simulink library "HWController_NGCHP_Genset_3p5MVA_lib"  (Simulink 8.1)
settings: Solver=ode45  StartTime=0.0  StopTime=10.0  RelTol=1e-3
undefined symbols (not defined in the file): Ts
libraries: HWController_NGCHP_Genset_3p5MVA_lib x2, powerlib x2, CHP_Model_lib x1, rtio_generic_modbus x1, simulink x1, GEJenbacherJ620_lib x1
settings Model: Creator=RE25624  LastModifiedBy=RE25624

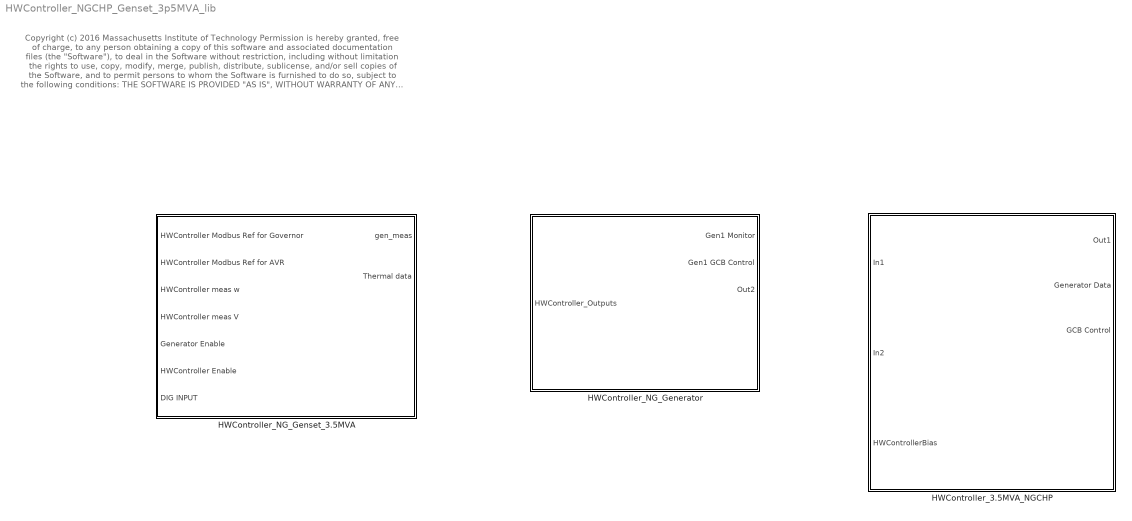
== system HWController_NGCHP_Genset_3p5MVA_lib ==
  note: Copyright (c) 2016 Massachusetts Institute of Technology
      | Permission is hereby granted, free of charge, to any person obtaining a copy of this software and associated documentation files (the "Software"), to deal
      | in the Software without restriction, including without limitation the rights to use, copy, modify, merge, publish, distribute, sublicense, and/or sell copies of the
      | Software, and to permit persons to whom the Software is furnished to do so, subject to the following conditions:
      |
      | THE SOFTWARE IS PROVIDED "AS IS", WITHOUT WARRANTY OF ANY KIND, EXPRESS OR IMPLIED, INCLUDING BUT NOT LIMITED TO THE
      | WARRANTIES OF MERCHANTABILITY, FITNESS FOR A PARTICULAR PURPOSE AND NONINFRINGEMENT. IN NO EVENT SHALL THE AUTHORS
      | OR COPYRIGHT HOLDERS BE LIABLE FOR ANY CLAIM, DAMAGES OR OTHER LIABILITY, WHETHER IN AN ACTION OF CONTRACT, TORT OR
      | OTHERWISE, ARISING FROM, OUT OF OR IN CONNECTION WITH THE SOFTWARE OR THE USE OR OTHER DEALINGS IN THE SOFTWARE
  HWController_3.5MVA_NGCHP : Subsystem
  HWController_NG_Generator : Subsystem
  HWController_NG_Genset_3.5MVA : Subsystem  mask(Gen-Set with simulated control modes){control_mode=1}
      mask prompts: control_mode "Control Mode [0 => Sim. 1 => Wood.]"
      mask help:
      | This Gen-Set block allows the user to indicate the control mode of the generator. The available control modes are: (1) PQ, (2) PV, and (3) VF.
      | The input values to the block will be applied according to the selected control mode.
      | For example, if PQ mode is selected, the controller will only work based on P_ref and Q_ref ignoring values of other inputs to the block.

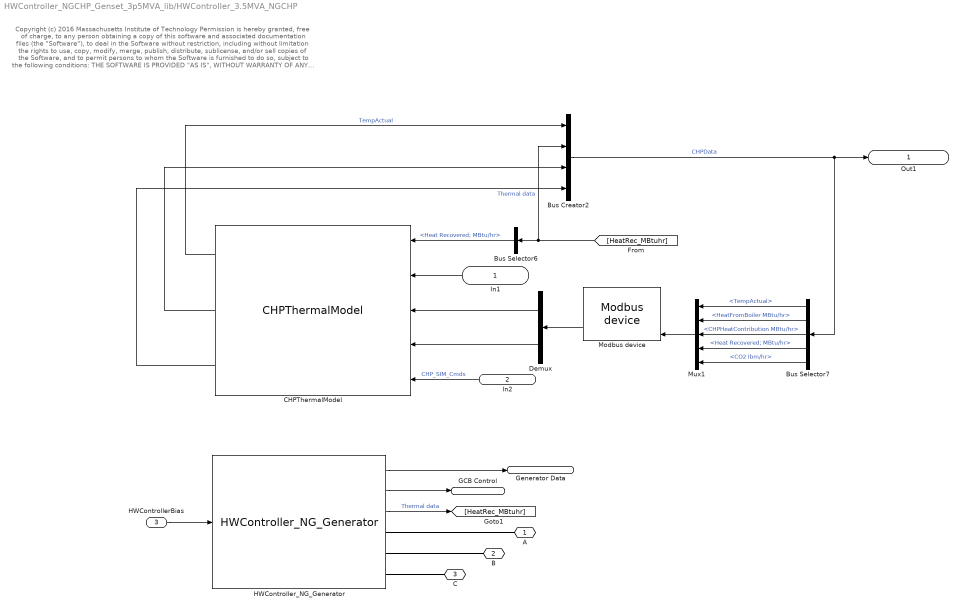
== system HWController_NGCHP_Genset_3p5MVA_lib/HWController_3.5MVA_NGCHP ==
  note: Copyright (c) 2016 Massachusetts Institute of Technology
      | Permission is hereby granted, free of charge, to any person obtaining a copy of this software and associated documentation files (the "Software"), to deal
      | in the Software without restriction, including without limitation the rights to use, copy, modify, merge, publish, distribute, sublicense, and/or sell copies of the
      | Software, and to permit persons to whom the Software is furnished to do so, subject to the following conditions:
      |
      | THE SOFTWARE IS PROVIDED "AS IS", WITHOUT WARRANTY OF ANY KIND, EXPRESS OR IMPLIED, INCLUDING BUT NOT LIMITED TO THE
      | WARRANTIES OF MERCHANTABILITY, FITNESS FOR A PARTICULAR PURPOSE AND NONINFRINGEMENT. IN NO EVENT SHALL THE AUTHORS
      | OR COPYRIGHT HOLDERS BE LIABLE FOR ANY CLAIM, DAMAGES OR OTHER LIABILITY, WHETHER IN AN ACTION OF CONTRACT, TORT OR
      | OTHERWISE, ARISING FROM, OUT OF OR IN CONNECTION WITH THE SOFTWARE OR THE USE OR OTHER DEALINGS IN THE SOFTWARE
  In1 : Inport
  In2 : Inport  Port=2
  HWControllerBias : Inport  Port=3
  Bus Creator2 : BusCreator
  Bus Selector6 : BusSelector  OutputSignals=Heat Recovered; MBtu/hr
  Bus Selector7 : BusSelector  OutputSignals=TempActual,HeatFromBoiler MBtu/hr,CHPHeatContribution MBtu/hr,Thermal data.Heat Recovered; MBtu/hr,Thermal data.CO2 lbm/hr
  CHPThermalModel : CHP_Model_lib/CHPThermalModel  SIM_HIL=SIM_HIL
  Demux : Demux  Outputs=2
  HWController_NG_Generator : HWController_NGCHP_Genset_3p5MVA_lib/HWController_NG_Generator
  Modbus device : rtio_generic_modbus/Modbus device  conf_name=CHP_slave_cfg.opal  conf_name_mask=CHP_slave_cfg.xls  sample_time=Ts
  Mux1 : Mux  Inputs=5
  A : PMIOPort  Tag=A  Port=1  Side=Right
      settings: AttributesFormatString=A
  B : PMIOPort  Port=2  Side=Right
  C : PMIOPort  Port=3  Side=Right
  Out1 : Outport
  Generator Data : Outport  Port=2
  GCB Control : Outport  Port=3
  wires:
  HWControllerBias/1 -> HWController_NG_Generator/1
  HWController_NG_Generator/3 -> [HeatRec_MBtuhr]  "Thermal data"
  Bus Selector7/3 -> Mux1/3  "<CHPHeatContribution MBtu/hr>"
  CHPThermalModel/1 -> Bus Creator2/1  "TempActual"
  Demux/2 -> CHPThermalModel/4
  CHPThermalModel/2 -> Bus Creator2/3
  Bus Selector7/2 -> Mux1/2  "<HeatFromBoiler MBtu/hr>"
  Bus Selector7/5 -> Mux1/5  "<CO2 lbm/hr>"
  Bus Selector7/4 -> Mux1/4  "<Heat Recovered; MBtu/hr>"
  Bus Selector7/1 -> Mux1/1  "<TempActual>"
  In1/1 -> CHPThermalModel/2
  Mux1/1 -> Modbus device/4
  Demux/1 -> CHPThermalModel/3
  CHPThermalModel/3 -> Bus Creator2/4
  [HeatRec_MBtuhr] -> Bus Creator2/2, Bus Selector6/1  "Thermal data"
  Modbus device/2 -> Demux/1
  HWController_NG_Generator/1 -> Generator Data/1
  HWController_NG_Generator/2 -> GCB Control/1
  Bus Selector6/1 -> CHPThermalModel/1  "<Heat Recovered; MBtu/hr>"
  Bus Creator2/1 -> Out1/1, Bus Selector7/1  "CHPData"
  In2/1 -> CHPThermalModel/5  "CHP_SIM_Cmds"
  connections:
  HWController_NG_Generator/RConn3 -- C/RConn1
  HWController_NG_Generator/RConn2 -- B/RConn1
  HWController_NG_Generator/RConn1 -- A/RConn1

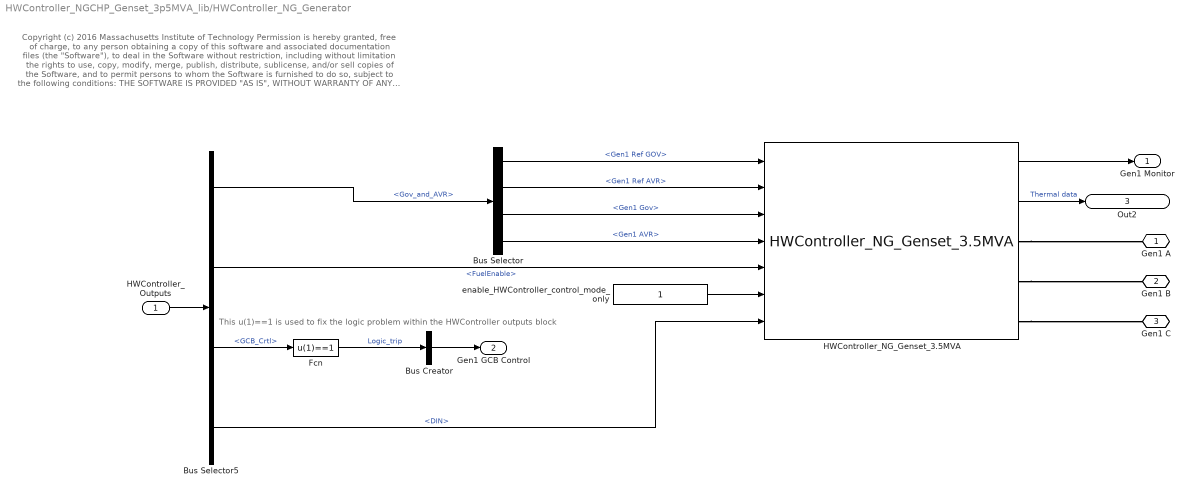
== system HWController_NGCHP_Genset_3p5MVA_lib/HWController_NG_Generator ==
  note: This u(1)==1 is used to fix the logic problem within the HWController outputs block
  note: Copyright (c) 2016 Massachusetts Institute of Technology
      | Permission is hereby granted, free of charge, to any person obtaining a copy of this software and associated documentation files (the "Software"), to deal
      | in the Software without restriction, including without limitation the rights to use, copy, modify, merge, publish, distribute, sublicense, and/or sell copies of the
      | Software, and to permit persons to whom the Software is furnished to do so, subject to the following conditions:
      |
      | THE SOFTWARE IS PROVIDED "AS IS", WITHOUT WARRANTY OF ANY KIND, EXPRESS OR IMPLIED, INCLUDING BUT NOT LIMITED TO THE
      | WARRANTIES OF MERCHANTABILITY, FITNESS FOR A PARTICULAR PURPOSE AND NONINFRINGEMENT. IN NO EVENT SHALL THE AUTHORS
      | OR COPYRIGHT HOLDERS BE LIABLE FOR ANY CLAIM, DAMAGES OR OTHER LIABILITY, WHETHER IN AN ACTION OF CONTRACT, TORT OR
      | OTHERWISE, ARISING FROM, OUT OF OR IN CONNECTION WITH THE SOFTWARE OR THE USE OR OTHER DEALINGS IN THE SOFTWARE
  HWController_Outputs : Inport
  Bus Creator : BusCreator  Inputs=1
  Bus Selector : BusSelector  OutputSignals=Gen1 Ref GOV,Gen1 Ref AVR,Gen1 Gov,Gen1 AVR
  Bus Selector5 : BusSelector  OutputSignals=Gov_and_AVR,FuelEnable,GCB_Crtl,DIN
  Fcn : Fcn  Expr=u(1)==1
  HWController_NG_Genset_3.5MVA : HWController_NGCHP_Genset_3p5MVA_lib/HWController_NG_Genset_3.5MVA  control_mode=1
  enable_HWController_control_mode_only : Constant
  Gen1 A : PMIOPort  Port=1  Side=Right
  Gen1 B : PMIOPort  Port=2  Side=Right
  Gen1 C : PMIOPort  Port=3  Side=Right
  Gen1 Monitor : Outport
  Gen1 GCB Control : Outport  Port=2
  Out2 : Outport  Port=3
  wires:
  Fcn/1 -> Bus Creator/1  "Logic_trip"
  Bus Creator/1 -> Gen1 GCB Control/1
  HWController_NG_Genset_3.5MVA/1 -> Gen1 Monitor/1
  enable_HWController_control_mode_only/1 -> HWController_NG_Genset_3.5MVA/6
  Bus Selector5/3 -> Fcn/1  "<GCB_Crtl>"
  HWController_NG_Genset_3.5MVA/2 -> Out2/1  "Thermal data"
  Bus Selector5/4 -> HWController_NG_Genset_3.5MVA/7  "<DIN>"
  Bus Selector5/1 -> Bus Selector/1  "<Gov_and_AVR>"
  HWController_Outputs/1 -> Bus Selector5/1
  Bus Selector5/2 -> HWController_NG_Genset_3.5MVA/5  "<FuelEnable>"
  Bus Selector/1 -> HWController_NG_Genset_3.5MVA/1  "<Gen1 Ref GOV>"
  Bus Selector/2 -> HWController_NG_Genset_3.5MVA/2  "<Gen1 Ref AVR>"
  Bus Selector/3 -> HWController_NG_Genset_3.5MVA/3  "<Gen1 Gov>"
  Bus Selector/4 -> HWController_NG_Genset_3.5MVA/4  "<Gen1 AVR>"
  connections:
  HWController_NG_Genset_3.5MVA/RConn1 -- Gen1 A/RConn1
  HWController_NG_Genset_3.5MVA/RConn2 -- Gen1 B/RConn1
  HWController_NG_Genset_3.5MVA/RConn3 -- Gen1 C/RConn1

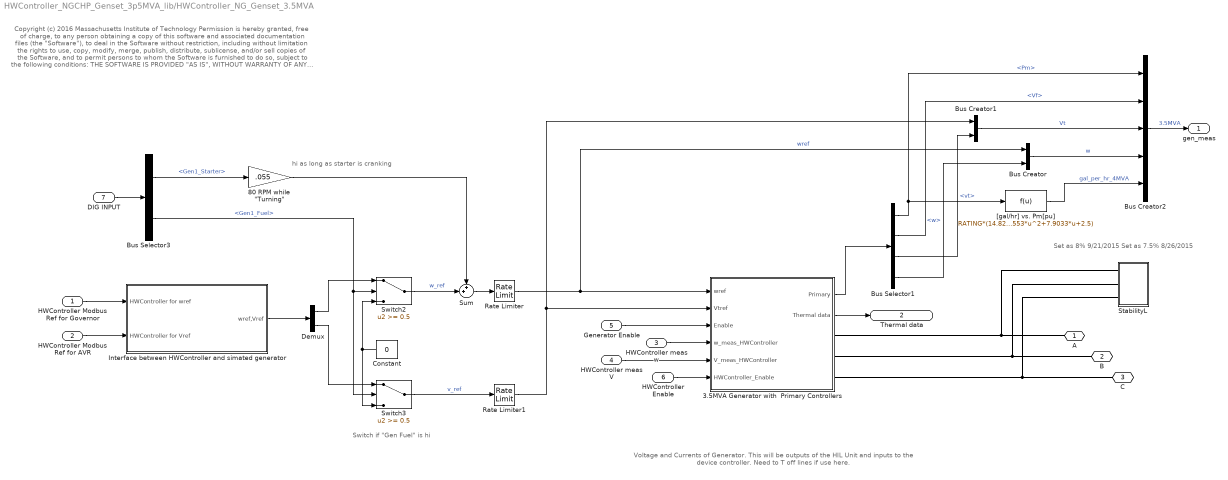
== system HWController_NGCHP_Genset_3p5MVA_lib/HWController_NG_Genset_3.5MVA ==
  note: Copyright (c) 2016 Massachusetts Institute of Technology
      | Permission is hereby granted, free of charge, to any person obtaining a copy of this software and associated documentation files (the "Software"), to deal
      | in the Software without restriction, including without limitation the rights to use, copy, modify, merge, publish, distribute, sublicense, and/or sell copies of the
      | Software, and to permit persons to whom the Software is furnished to do so, subject to the following conditions:
      |
      | THE SOFTWARE IS PROVIDED "AS IS", WITHOUT WARRANTY OF ANY KIND, EXPRESS OR IMPLIED, INCLUDING BUT NOT LIMITED TO THE
      | WARRANTIES OF MERCHANTABILITY, FITNESS FOR A PARTICULAR PURPOSE AND NONINFRINGEMENT. IN NO EVENT SHALL THE AUTHORS
      | OR COPYRIGHT HOLDERS BE LIABLE FOR ANY CLAIM, DAMAGES OR OTHER LIABILITY, WHETHER IN AN ACTION OF CONTRACT, TORT OR
      | OTHERWISE, ARISING FROM, OUT OF OR IN CONNECTION WITH THE SOFTWARE OR THE USE OR OTHER DEALINGS IN THE SOFTWARE
  note: hi as long as starter is cranking
  note: Switch if "Gen Fuel" is hi
  note: Voltage and Currents of Generator.
      | This will be outputs of the HIL Unit
      | and inputs to the device controller.
      | Need to T off lines if use here.
  note: Set as 8% 9/21/2015
      | Set as 7.5% 8/26/2015
  HWController Modbus Ref for Governor : Inport
  HWController Modbus Ref for AVR : Inport  Port=2
  HWController meas w : Inport  Port=3
  HWController meas V : Inport  Port=4
  Generator Enable : Inport  Port=5
  HWController Enable : Inport  Port=6
  DIG INPUT : Inport  Port=7
  3.5MVA Generator with  Primary Controllers : Subsystem
  "80 RPM while \"Turning\"" : Gain  Gain=.055
  Bus Creator : BusCreator  Inputs=2
  Bus Creator1 : BusCreator  Inputs=2
  Bus Creator2 : BusCreator  Inputs=5
  Bus Selector1 : BusSelector  OutputSignals=Pm,Vf,vt,w
  Bus Selector3 : BusSelector  OutputSignals=DIN.DI_CH00-07.Gen1_Starter,DIN.DI_CH00-07.Gen1_Fuel
  Constant : Constant  Value=0
  Demux : Demux  Outputs=2
  Interface between HWController and simated generator : Subsystem
  Rate Limiter : RateLimiter  RisingSlewLimit=0.5  FallingSlewLimit=-0.5  SampleTimeMode=inherited
  Rate Limiter1 : RateLimiter  RisingSlewLimit=0.5  FallingSlewLimit=-0.5  SampleTimeMode=inherited
  StabilityL : Subsystem  mask{v=13800, kVA=320, pf=1}
  Sum : Sum  Inputs=++|
  Switch2 : Switch  Threshold=0.5
  Switch3 : Switch  Threshold=0.5
  "[gal/hr] vs. Pm[pu]" : Fcn  Expr=RATING*(14.827*u^4-27.253*u^3+15.553*u^2+7.9033*u+2.5)  mask{RATING=4}
      mask prompts: RATING "Rating [MW]"
      mask help: This block computes the gal/hr vs Pm[pu] of a generator of a given rating [MW].
  A : PMIOPort  Port=1  Side=Right
  B : PMIOPort  Port=2  Side=Right
  C : PMIOPort  Port=3  Side=Right
  gen_meas : Outport
  Thermal data : Outport  Port=2
  wires:
  HWController Enable/1 -> 3.5MVA Generator with  Primary Controllers/6(HWController_Enable)
  HWController meas V/1 -> 3.5MVA Generator with  Primary Controllers/5(V_meas_HWController)
  HWController meas w/1 -> 3.5MVA Generator with  Primary Controllers/4(w_meas_HWController)
  Interface between HWController and simated generator/1(wref,Vref) -> Demux/1
  HWController Modbus Ref for Governor/1 -> Interface between HWController and simated generator/1(HWController for wref)
  HWController Modbus Ref for AVR/1 -> Interface between HWController and simated generator/2(HWController for Vref)
  3.5MVA Generator with  Primary Controllers/1(Primary) -> Bus Selector1/1
  Switch2/1 -> Sum/2  "w_ref"
  Demux/1 -> Switch2/1
  Demux/2 -> Switch3/1
  Constant/1 -> Switch3/3, Switch2/3
  Switch3/1 -> Rate Limiter1/1  "v_ref"
  Bus Selector1/3 -> Bus Creator1/2  "<vt>"
  Bus Selector1/2 -> Bus Creator2/2  "<Vf>"
  Bus Selector1/1 -> Bus Creator2/1, "[gal/hr] vs. Pm[pu]"/1  "<Pm>"
  Bus Creator1/1 -> Bus Creator2/3  "Vt"
  Bus Creator/1 -> Bus Creator2/4  "w"
  Bus Creator2/1 -> gen_meas/1  "3.5MVA"
  Rate Limiter/1 -> 3.5MVA Generator with  Primary Controllers/1(wref), Bus Creator/1  "wref"
  Rate Limiter1/1 -> 3.5MVA Generator with  Primary Controllers/2(Vtref), Bus Creator1/1
  "[gal/hr] vs. Pm[pu]"/1 -> Bus Creator2/5  "gal_per_hr_4MVA"
  3.5MVA Generator with  Primary Controllers/2(Thermal data) -> Thermal data/1
  Bus Selector1/4 -> Bus Creator/2  "<w>"
  DIG INPUT/1 -> Bus Selector3/1
  Sum/1 -> Rate Limiter/1
  "80 RPM while \"Turning\""/1 -> Sum/1
  Bus Selector3/1 -> "80 RPM while \"Turning\""/1  "<Gen1_Starter>"
  Bus Selector3/2 -> Switch3/2, Switch2/2  "<Gen1_Fuel>"
  Generator Enable/1 -> 3.5MVA Generator with  Primary Controllers/3(Enable)
  connections:
  StabilityL/LConn1 -- 3.5MVA Generator with  Primary Controllers/RConn1 -- A/RConn1
  StabilityL/LConn2 -- B/RConn1 -- 3.5MVA Generator with  Primary Controllers/RConn2
  StabilityL/LConn3 -- 3.5MVA Generator with  Primary Controllers/RConn3 -- C/RConn1

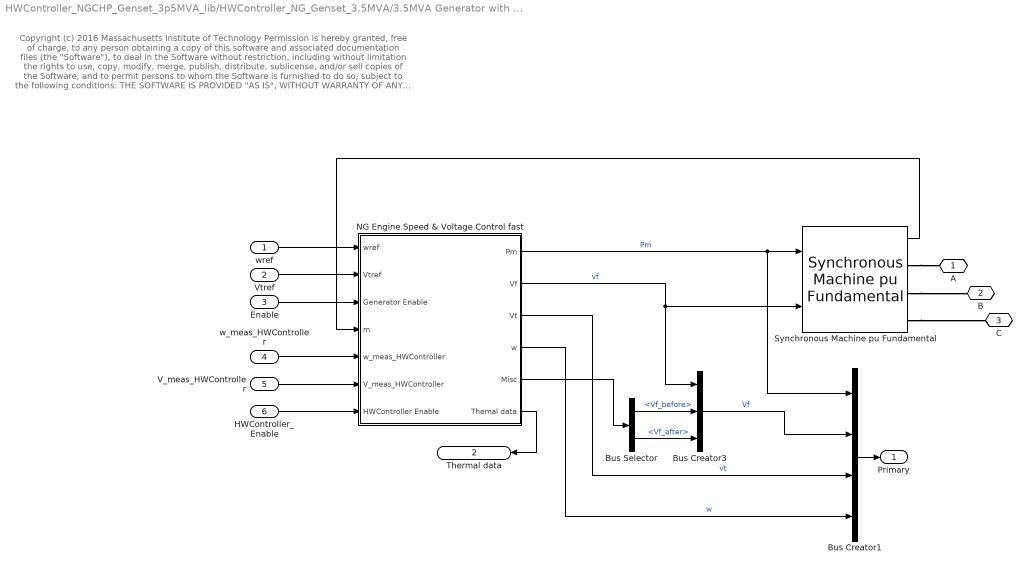
== system HWController_NGCHP_Genset_3p5MVA_lib/HWController_NG_Genset_3.5MVA/3.5MVA Generator with  Primary Controllers ==
  note: Copyright (c) 2016 Massachusetts Institute of Technology
      | Permission is hereby granted, free of charge, to any person obtaining a copy of this software and associated documentation files (the "Software"), to deal
      | in the Software without restriction, including without limitation the rights to use, copy, modify, merge, publish, distribute, sublicense, and/or sell copies of the
      | Software, and to permit persons to whom the Software is furnished to do so, subject to the following conditions:
      |
      | THE SOFTWARE IS PROVIDED "AS IS", WITHOUT WARRANTY OF ANY KIND, EXPRESS OR IMPLIED, INCLUDING BUT NOT LIMITED TO THE
      | WARRANTIES OF MERCHANTABILITY, FITNESS FOR A PARTICULAR PURPOSE AND NONINFRINGEMENT. IN NO EVENT SHALL THE AUTHORS
      | OR COPYRIGHT HOLDERS BE LIABLE FOR ANY CLAIM, DAMAGES OR OTHER LIABILITY, WHETHER IN AN ACTION OF CONTRACT, TORT OR
      | OTHERWISE, ARISING FROM, OUT OF OR IN CONNECTION WITH THE SOFTWARE OR THE USE OR OTHER DEALINGS IN THE SOFTWARE
  wref : Inport
  Vtref : Inport  Port=2
  Enable : Inport  Port=3
  w_meas_HWController : Inport  Port=4
  V_meas_HWController : Inport  Port=5
  HWController_Enable : Inport  Port=6
  Bus Creator1 : BusCreator
  Bus Creator3 : BusCreator  Inputs=3
  Bus Selector : BusSelector  OutputSignals=Vf_before,Vf_after
  NG Engine Speed & Voltage Control fast : Subsystem
  Synchronous Machine pu Fundamental : powerlib/Machines/Synchronous Machine pu Fundamental  PresetModel=No  MechanicalLoad=Mechanical power Pm  ShowDetailedParameters=on  RotorType=Salient-pole  NominalParameters=[3.5e+006 13800 60]  Stator=[0.008979 0.05 2.35 1.72]  Field=[0.00206 0.511]  Dampers2=[0.0652, 0.5134, 0.0287, 0.2553, 7.765e-3, 0.9167 ]  Dampers1=[0.2826 3.738 0.02545 0.2392]  Mechanical=[0.3468 0.009238 2]  PolePairs=2  InitialConditions="[ -99  0  0  0  0  0  0  0  0 ]"  SetSaturation=off  Saturation=[0.6404,0.7127,0.8441,0.9214,0.9956,1.082,1.19,1.316,1.457;0.7,0.7698,0.8872,0.9466,0.9969,1.046,1.1,1.151,1.201]  Units=per unit fundamental parameters  LoadFlowParameters=[1,0,0,0,0]  TsPowergui=0  TsBlock=-1  IterativeModel=Forward Euler  BusType=swing  Pref=0  Qref=0  Qmin=-inf  Qmax=inf  PLF=0  QLF=0
  A : PMIOPort  Port=1  Side=Right
  B : PMIOPort  Port=2  Side=Right
  C : PMIOPort  Port=3  Side=Right
  Primary : Outport
  Thermal data : Outport  Port=2
  wires:
  HWController_Enable/1 -> NG Engine Speed & Voltage Control fast/7(HWController Enable)
  Bus Creator3/1 -> Bus Creator1/2  "Vf"
  Bus Selector/2 -> Bus Creator3/3  "<Vf_after>"
  Bus Selector/1 -> Bus Creator3/2  "<Vf_before>"
  NG Engine Speed & Voltage Control fast/5(Misc) -> Bus Selector/1
  Bus Creator1/1 -> Primary/1
  NG Engine Speed & Voltage Control fast/4(w) -> Bus Creator1/4  "w"
  NG Engine Speed & Voltage Control fast/3(Vt) -> Bus Creator1/3  "vt"
  V_meas_HWController/1 -> NG Engine Speed & Voltage Control fast/6(V_meas_HWController)
  w_meas_HWController/1 -> NG Engine Speed & Voltage Control fast/5(w_meas_HWController)
  Synchronous Machine pu Fundamental/1 -> NG Engine Speed & Voltage Control fast/4(m)
  Enable/1 -> NG Engine Speed & Voltage Control fast/3(Generator Enable)
  NG Engine Speed & Voltage Control fast/1(Pm) -> Synchronous Machine pu Fundamental/1, Bus Creator1/1  "Pm"
  NG Engine Speed & Voltage Control fast/2(Vf) -> Synchronous Machine pu Fundamental/2, Bus Creator3/1  "vf"
  wref/1 -> NG Engine Speed & Voltage Control fast/1(wref)
  Vtref/1 -> NG Engine Speed & Voltage Control fast/2(Vtref)
  NG Engine Speed & Voltage Control fast/6(Themal data) -> Thermal data/1
  connections:
  Synchronous Machine pu Fundamental/RConn1 -- A/RConn1
  Synchronous Machine pu Fundamental/RConn2 -- B/RConn1
  Synchronous Machine pu Fundamental/RConn3 -- C/RConn1

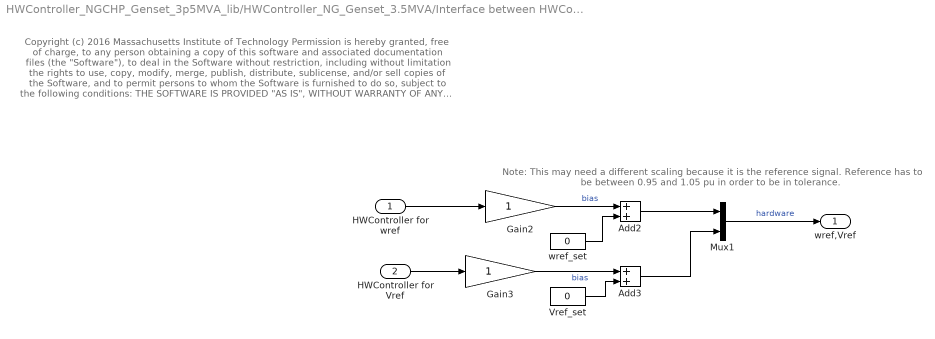
== system HWController_NGCHP_Genset_3p5MVA_lib/HWController_NG_Genset_3.5MVA/Interface between HWController and simated generator ==
  note: Copyright (c) 2016 Massachusetts Institute of Technology
      | Permission is hereby granted, free of charge, to any person obtaining a copy of this software and associated documentation files (the "Software"), to deal
      | in the Software without restriction, including without limitation the rights to use, copy, modify, merge, publish, distribute, sublicense, and/or sell copies of the
      | Software, and to permit persons to whom the Software is furnished to do so, subject to the following conditions:
      |
      | THE SOFTWARE IS PROVIDED "AS IS", WITHOUT WARRANTY OF ANY KIND, EXPRESS OR IMPLIED, INCLUDING BUT NOT LIMITED TO THE
      | WARRANTIES OF MERCHANTABILITY, FITNESS FOR A PARTICULAR PURPOSE AND NONINFRINGEMENT. IN NO EVENT SHALL THE AUTHORS
      | OR COPYRIGHT HOLDERS BE LIABLE FOR ANY CLAIM, DAMAGES OR OTHER LIABILITY, WHETHER IN AN ACTION OF CONTRACT, TORT OR
      | OTHERWISE, ARISING FROM, OUT OF OR IN CONNECTION WITH THE SOFTWARE OR THE USE OR OTHER DEALINGS IN THE SOFTWARE
  note: Note: This may need a different scaling because it is the reference signal.
      | Reference has to be between 0.95 and 1.05 pu in order to be in tolerance.
  HWController for wref : Inport
  HWController for Vref : Inport  Port=2
  Add2 : Sum
  Add3 : Sum
  Gain2 : Gain
  Gain3 : Gain
  Mux1 : Mux  Inputs=2
  Vref_set : Constant  Value=0
  wref_set : Constant  Value=0
  wref,Vref : Outport
  wires:
  Gain2/1 -> Add2/1  "bias"
  Add2/1 -> Mux1/1
  Gain3/1 -> Add3/1  "bias"
  Vref_set/1 -> Add3/2
  Add3/1 -> Mux1/2
  HWController for wref/1 -> Gain2/1
  Mux1/1 -> wref,Vref/1  "hardware"
  HWController for Vref/1 -> Gain3/1
  wref_set/1 -> Add2/2

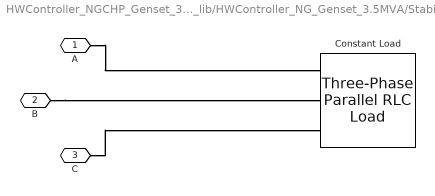
== system HWController_NGCHP_Genset_3p5MVA_lib/HWController_NG_Genset_3.5MVA/StabilityL ==
  Constant Load : powerlib/Elements/Three-Phase Parallel RLC Load  LConnTagsString=A|B|C  Configuration=Y (grounded)  NominalVoltage=v  NominalFrequency=60  ActivePower=kVA*1E3*pf  InductivePower=kVA*1E3*sqrt(1-pf^2)  CapacitivePower=0  Measurements=None  LoadType=constant Z
  A : PMIOPort  Port=1  Side=Left
  B : PMIOPort  Port=2  Side=Left
  C : PMIOPort  Port=3  Side=Left
  connections:
  A/RConn1 -- Constant Load/LConn1
  B/RConn1 -- Constant Load/LConn2
  C/RConn1 -- Constant Load/LConn3

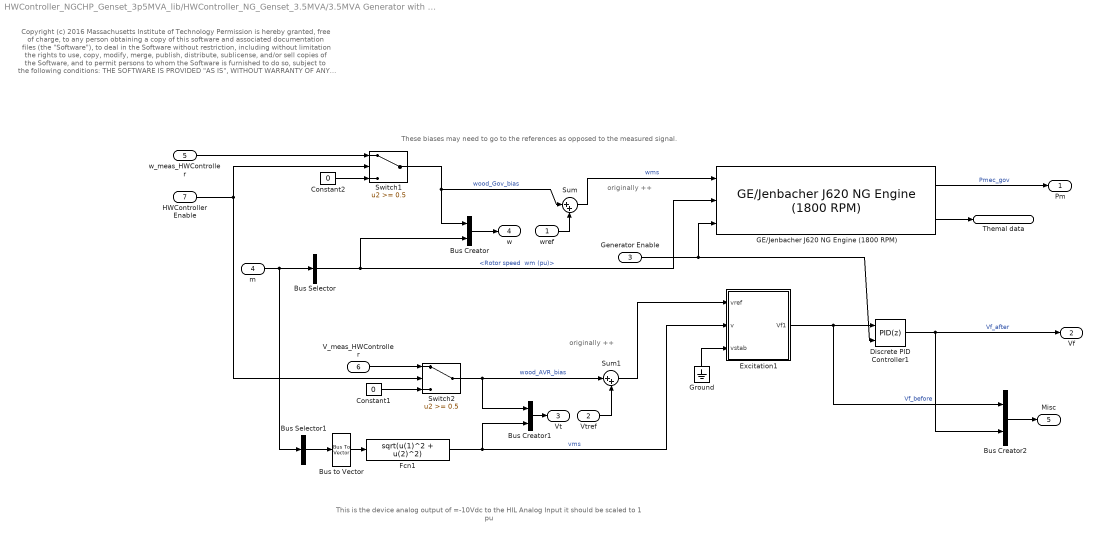
== system HWController_NGCHP_Genset_3p5MVA_lib/HWController_NG_Genset_3.5MVA/3.5MVA Generator with  Primary Controllers/NG Engine Speed & Voltage Control fast ==
  note: Copyright (c) 2016 Massachusetts Institute of Technology
      | Permission is hereby granted, free of charge, to any person obtaining a copy of this software and associated documentation files (the "Software"), to deal
      | in the Software without restriction, including without limitation the rights to use, copy, modify, merge, publish, distribute, sublicense, and/or sell copies of the
      | Software, and to permit persons to whom the Software is furnished to do so, subject to the following conditions:
      |
      | THE SOFTWARE IS PROVIDED "AS IS", WITHOUT WARRANTY OF ANY KIND, EXPRESS OR IMPLIED, INCLUDING BUT NOT LIMITED TO THE
      | WARRANTIES OF MERCHANTABILITY, FITNESS FOR A PARTICULAR PURPOSE AND NONINFRINGEMENT. IN NO EVENT SHALL THE AUTHORS
      | OR COPYRIGHT HOLDERS BE LIABLE FOR ANY CLAIM, DAMAGES OR OTHER LIABILITY, WHETHER IN AN ACTION OF CONTRACT, TORT OR
      | OTHERWISE, ARISING FROM, OUT OF OR IN CONNECTION WITH THE SOFTWARE OR THE USE OR OTHER DEALINGS IN THE SOFTWARE
  note: originally ++
  note: originally ++
  note: These biases may need to
      | go to the references as opposed
      | to the measured signal.
  note: This is the device analog output of =-10Vdc to
      | the HIL Analog Input it should be scaled to 1 pu
  wref : Inport  SampleTime=Ts
  Vtref : Inport  Port=2  SampleTime=Ts
  Generator Enable : Inport  Port=3  SampleTime=Ts
  m : Inport  Port=4  SampleTime=Ts
  w_meas_HWController : Inport  Port=5  SampleTime=Ts
  V_meas_HWController : Inport  Port=6  SampleTime=Ts
  HWController Enable : Inport  Port=7  SampleTime=Ts
  Bus Creator : BusCreator  Inputs=2
  Bus Creator1 : BusCreator  Inputs=2
  Bus Creator2 : BusCreator  Inputs=2
  Bus Selector : BusSelector  OutputSignals="Mechanical.Rotor speed  wm (pu)"
  Bus Selector1 : BusSelector  OutputSignals="dq0 components.Stator voltage  vd (pu),dq0 components.Stator voltage  vq (pu)"  OutputAsBus=on
  Bus to Vector : BusToVector
  Constant1 : Constant  Value=0
  Constant2 : Constant  Value=0
  Discrete PID Controller1 : simulink/Continuous/PID Controller  Controller=PID  TimeDomain=Discrete-time  SampleTime=-1  IntegratorMethod=Forward Euler  FilterMethod=Forward Euler  Form=Parallel  P=1  I=0  D=0  N=100  InitialConditionSource=internal  InitialConditionForIntegrator=0  InitialConditionForFilter=0  ExternalReset=either  LimitOutput=on  UpperSaturationLimit=5  LowerSaturationLimit=-5  LinearizeAsGain=off  AntiWindupMode=none  Kb=1  TrackingMode=off  Kt=1  PParamMin=[]  PParamMax=[]  IParamMin=[]  IParamMax=[]  DParamMin=[]  DParamMax=[]  NParamMin=[]  NParamMax=[]  KbParamMin=[]  KbParamMax=[]  KtParamMin=[]  KtParamMax=[]  POutMin=[]  POutMax=[]  IOutMin=[]  IOutMax=[]  DOutMin=[]  DOutMax=[]  NOutMin=[]  NOutMax=[]  KbOutMin=[]  KbOutMax=[]  KtOutMin=[]  KtOutMax=[]  IntegratorOutMin=[]  IntegratorOutMax=[]  FilterOutMin=[]  FilterOutMax=[]  SumOutMin=[]  SumOutMax=[]  SumI1OutMin=[]  SumI1OutMax=[]  SumI2OutMin=[]  SumI2OutMax=[]  SumI3OutMin=[]  SumI3OutMax=[]  SumDOutMin=[]  SumDOutMax=[]  SaturationOutMin=[]  SaturationOutMax=[]  IntegratorContinuousStateAttributes=''  IntegratorStateMustResolveToSignalObject=off  IntegratorRTWStateStorageClass=Auto  FilterContinuousStateAttributes=''  FilterStateMustResolveToSignalObject=off  FilterRTWStateStorageClass=Auto
  Excitation1 : Subsystem  mask(Excitation System){tr=20e-4, reg=[ 200 2e-3 ], exc=[ 1 0.00000001 ], tgr=[ 1e-12 1e-12 ], damp=[0 1e-12 ], sat=[], lim=[ 0 5 0 ], v0=[ 0 0 ]}
      mask prompts: tr "Low-pass filter time constant Tr:"; reg "Regulator gain and time constant [ Ka  Ta ]:"; exc "Exciter  [ Ke  Te ]:"; tgr "Transient gain reduction [ Tb  Tc ]:"; damp "Damping filter gain and time constant  [ Kf  Tf  ]:"; sat "Field saturation parameters [ A B ]:"; lim "Regulator output limits and gain [ Efmin  Efmax  Kp ]:"; v0 "Initial values of terminal voltage  and field voltage [ Vt0 Vf0 ] :"
      mask help:
      | Implements an IEEE type 1 synchronous machine voltage regulator combined
      | to an exciter.
      |
      | The output of the block is the field voltage vfd, in pu,  to be applied to the Vf
      | Simulink input of a Synchronous Machine block.
      |
      | Connect the Vd and Vq measurements signals of the Synchronous Machine block
      | (signals 9 and 10)  to  the Vd and Vq inputs of the Excitation System block.
      mask Help: helpview(psbhelp);
  Fcn1 : Fcn  Expr=sqrt(u(1)^2 + u(2)^2)
  GE/Jenbacher J620 NG Engine (1800 RPM) : GEJenbacherJ620_lib/GE//Jenbacher J620 NG Engine (1800 RPM)  cd=.8  H=47133  keq=1.3962  Ma=.029  Meq=.0285  Mf=.019  P0=800000  Pm=37241  R=8.314  T0=300  Tm=325  thermalEfficiency=.45  V=0.031  Vd=0.125  volumeEfficiency=.9  P=3  I=3  UL=1.05  LL=0  UPL=1.5  LPL=-1.5
  Ground : Ground
  Sum : Sum  Inputs=|++
  Sum1 : Sum  Inputs=|++
  Switch1 : Switch  Threshold=0.5
  Switch2 : Switch  Threshold=0.5
  Pm : Outport
  Vf : Outport  Port=2
  Vt : Outport  Port=3
  w : Outport  Port=4
  Misc : Outport  Port=5
  Themal data : Outport  Port=6
  wires:
  wref/1 -> Sum/2
  Sum/1 -> GE/Jenbacher J620 NG Engine (1800 RPM)/1  "wms"
  Sum1/1 -> Excitation1/1(vref)
  Vtref/1 -> Sum1/2
  Switch2/1 -> Bus Creator1/1, Sum1/1  "wood_AVR_bias"
  Constant1/1 -> Switch2/3
  Constant2/1 -> Switch1/3
  w_meas_HWController/1 -> Switch1/1
  Switch1/1 -> Sum/1, Bus Creator/1  "wood_Gov_bias"
  HWController Enable/1 -> Switch2/2, Switch1/2
  Bus Creator2/1 -> Misc/1
  Discrete PID Controller1/1 -> Bus Creator2/2, Vf/1  "Vf_after"
  Excitation1/1(Vf1) -> Bus Creator2/1, Discrete PID Controller1/1  "Vf_before"
  Bus Creator1/1 -> Vt/1
  Bus Creator/1 -> w/1
  Ground/1 -> Excitation1/3(vstab)
  Fcn1/1 -> Excitation1/2(v), Bus Creator1/2  "vms"
  V_meas_HWController/1 -> Switch2/1
  m/1 -> Bus Selector1/1, Bus Selector/1
  Bus Selector1/1 -> Bus to Vector/1
  Bus to Vector/1 -> Fcn1/1
  Generator Enable/1 -> GE/Jenbacher J620 NG Engine (1800 RPM)/3, Discrete PID Controller1/2
  GE/Jenbacher J620 NG Engine (1800 RPM)/1 -> Pm/1  "Pmec_gov"
  GE/Jenbacher J620 NG Engine (1800 RPM)/2 -> Themal data/1
  Bus Selector/1 -> GE/Jenbacher J620 NG Engine (1800 RPM)/2, Bus Creator/2  "<Rotor speed  wm (pu)>"

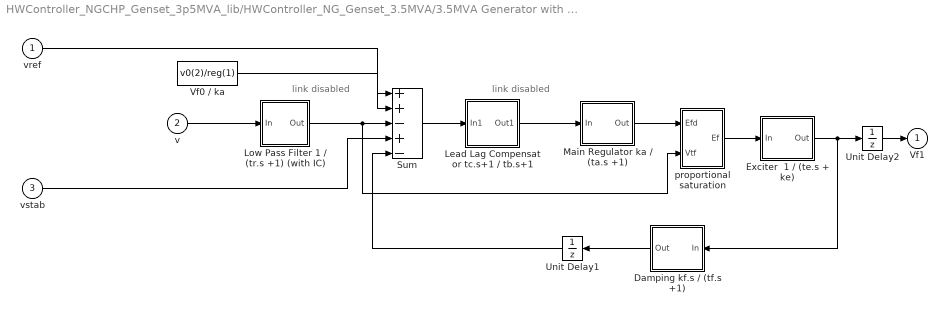
== system HWController_NGCHP_Genset_3p5MVA_lib/HWController_NG_Genset_3.5MVA/3.5MVA Generator with  Primary Controllers/NG Engine Speed & Voltage Control fast/Excitation1 ==
  note: link disabled
  note: link disabled
  vref : Inport
  v : Inport  Port=2
  vstab : Inport  Port=3
  Damping kf.s / (tf.s +1) : Subsystem
  Exciter  1 / (te.s + ke) : Subsystem
  Lead Lag Compensator tc.s+1 / tb.s+1 : Subsystem  AncestorBlock=|  mask(Discrete Lead-Lag Controller){T1=tgr(2), T2=tgr(1), V_Init=exc(1)*v0(2)/reg(1), Ts=Ts}
      | powerlib_extras/Discrete 
      | Control Blocks/Discrete
      | Lead-Lag
      mask prompts: T1 "Time constant T1 (s):"; T2 "Time constant T2 (s):"; V_Init "Initial input and output:"; Ts "Sample time (s):"
      mask help:
      | This block implements a discrete lead-lag controller:
      |
      |          1+T1s
      | H(s)= ------
      |          1+T2s
      |
      | States are initialized according to initial input anf output value so that simulation starts in steady state.
      mask init:
      | numc=[T1 1];
      | denc=[T2 1];
      | [Ac,Bc,Cc,Dc]=tf2ss(numc,denc);
      | 
      | %  Conversion to discrete transfer function
      | nstates = size(Ac,1);
      | invexp = inv(eye(nstates) - (Ts/2)*Ac);
      | Ad = invexp*(eye(nstates) + (Ts/2)*Ac);
      | Bd = invexp*Bc;
      | Cd = Cc*invexp*Ts;
      | Dd = Cc*invexp*Bc*(Ts/2) + Dc;
      | %
      | % Compute Initial states
      | I=eye(size(Ac));
      | x0c=inv(-Ac)*Bc*V_Init;
      | x0d=(I-Ac*Ts/2)*x0c/Ts - Bc/2*V_Init;
      | 
      | if T1==0 & T2==0, Dd=1; end
      mask Display: disp('1+T1s\n---\n1+T2s')
  Low Pass Filter 1 / (tr.s +1) (with IC) : Subsystem  AncestorBlock=|  mask(Discrete 1st-Order Filter){FilterType=Lowpass, Tc=tr, Ts=Ts, Initialize=on, Vac_Init=[0 0 60], Vdc_Init=v0(1), PlotResponse=off, param1=[1 500 0.1]}
      | powerlib_extras/Discrete 
      | Control Blocks/Discrete
      | 1st-Order
      | Discrete Filter
      mask prompts: FilterType "Filter Type:"; Tc "Time constant (s):"; Ts "Sample time:"; Initialize "Initialize filter states"; Vac_Init "AC initial input: [ Mag  Phase(degrees)  Freq(Hz) ]"; Vdc_Init "DC Initial input:"; PlotResponse "Plot filter response"; param1 "Frequency range(Hz) : [Start  End  Inc.]"
      mask init:
      | switch FilterType
      | case 1, % Lowpass
      |     X=[0 1 2 3 4];
      |     Y=[-2 -2 -3 -4 -4];
      |     numc=1;
      |     denc=[Tc 1];
      | case 2,   % Highpass
      |     X=[0 1 2 3 4];
      |     Y=[-4 -4 -3 -2 -2];
      |     numc=[1 0];
      |     denc=[1 1/Tc];
      | end
      | %
      | [Ac,Bc,Cc,Dc]=tf2ss(numc,denc);
      | %
      | %  Conversion to discrete transfer function
      | nstates = size(Ac,1);
      | invexp = inv(eye(nstates) - (Ts/2)*Ac);
      | Ad = invexp*(eye(nstates) + (Ts/2)*Ac);
      | Bd = invexp*Bc;
      | Cd = Cc*invexp*Ts;
      | Dd = Cc*invexp*Bc*(Ts/2) + Dc;
      | %
      | if Initialize==1  % Compute initial conditions on states
      |     u1=Vac_Init(1)*exp(j*Vac_Init(2)*pi/180);
      |     u2=Vdc_Init*exp(j*90*pi/180);
      |     u=u1+u2;
      |     u0=imag(u); % input at  t=0;
      |     I=eye(size(Ac));
      |     sI1=I*j*(2*pi*Vac_Init(3));
      |     sI2=I*j*0;
      |     x=inv(sI1-Ac)*Bc*u1 + inv(sI2-Ac)*Bc*u2;
      |     x0c=imag(x);
      |     x0d=(I-Ac*Ts/2)*x0c/Ts - Bc/2*u0;
      | else
      |     x0d=0;
      | end
      | 
      | %
      | if PlotResponse==1 % Plot frequency and step response
      |     figure(1)
      |     sys=ss(Ad,Bd,Cd,Dd,Ts);
      |     f=param1(1):param1(3):param1(2);
      |     w=2*pi*f;
      |     [mag phase]=bode(sys,w);
      |     subplot(2,1,1)
      |     plot(f,squeeze(mag))
      |     title('Magnitude')
      |     grid
      |     subplot(2,1,2)
      |     plot(f,squeeze(phase))
      |     title('Phase (degrees)')
      |     xlabel('Hz')
      |     grid
      |     figure(2)
      |     step(sys)
      | end
      mask TypeOptions FilterType: Lowpass | Highpass
      mask Callback Initialize: p4=get_param(gcb,'Initialize');if strcmp(p4,'on');visible={'on','on','on','on','on','on','on',get_param(gcb,'PlotResponse')};else;visible={'on','on','on','on','off','off','on',get_param(gcb,'PlotResponse')};end;set_param(gcb,'MaskVisibilities',visible)
      mask Callback PlotResponse: p7=get_param(gcb,'PlotResponse');if strcmp(p7,'on');visible={'on','on','on','on',get_param(gcb,'Initialize'),get_param(gcb,'Initialize'),'on','on'};else;visible={'on','on','on','on',get_param(gcb,'Initialize'),get_param(gcb,'Initialize'),'on','off'};end;set_param(gcb,'MaskVisibilities',visible)
      mask Display: plot(X,Y);
  Main Regulator ka / (ta.s +1) : Subsystem
  Sum : Sum  Inputs=++-+-  SaturateOnIntegerOverflow=on  InputSameDT=on  OutDataTypeStr=Inherit: Same as first input
  Unit Delay1 : UnitDelay  SampleTime=Ts
  Unit Delay2 : UnitDelay  InitialCondition=v0(2)  SampleTime=Ts
  Vf0 / ka : Constant  Value=v0(2)/reg(1)
  proportional saturation : Subsystem
  Vf1 : Outport  InitialOutput=0
  wires:
  Exciter  1 / (te.s + ke)/1(Out) -> Damping kf.s / (tf.s +1)/1(In), Unit Delay2/1
  Damping kf.s / (tf.s +1)/1(Out) -> Unit Delay1/1
  Main Regulator ka / (ta.s +1)/1(Out) -> proportional saturation/1(Efd)
  Vf0 / ka/1 -> Sum/2
  Low Pass Filter 1 / (tr.s +1) (with IC)/1(Out) -> Sum/3, proportional saturation/2(Vtf)
  vstab/1 -> Sum/4
  vref/1 -> Sum/1
  v/1 -> Low Pass Filter 1 / (tr.s +1) (with IC)/1(In)
  Sum/1 -> Lead Lag Compensator tc.s+1 / tb.s+1/1(In1)
  Lead Lag Compensator tc.s+1 / tb.s+1/1(Out1) -> Main Regulator ka / (ta.s +1)/1(In)
  proportional saturation/1(Ef) -> Exciter  1 / (te.s + ke)/1(In)
  Unit Delay1/1 -> Sum/5
  Unit Delay2/1 -> Vf1/1

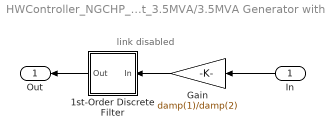
== system HWController_NGCHP_Genset_3p5MVA_lib/HWController_NG_Genset_3.5MVA/3.5MVA Generator with  Primary Controllers/NG Engine Speed & Voltage Control fast/Excitation1/Damping kf.s / (tf.s +1) ==
  note: link disabled
  In : Inport
  1st-Order Discrete Filter : Subsystem  AncestorBlock=|  mask(Discrete 1st-Order Filter){FilterType=Highpass, Tc=damp(2), Ts=Ts, Initialize=on, Vac_Init=[0 0 60], Vdc_Init=damp(1)*v0(2)/damp(2), PlotResponse=off, param1=[1 500 0.1]}
      | powerlib_extras/Discrete 
      | Control Blocks/Discrete
      | 1st-Order
      | Discrete Filter
      mask prompts: FilterType "Filter Type:"; Tc "Time constant (s):"; Ts "Sample time:"; Initialize "Initialize filter states"; Vac_Init "AC initial input: [ Mag  Phase(degrees)  Freq(Hz) ]"; Vdc_Init "DC Initial input:"; PlotResponse "Plot filter response"; param1 "Frequency range(Hz) : [Start  End  Inc.]"
      mask init: same as HWController_NGCHP_Genset_3p5MVA_lib/HWController_NG_Genset_3.5MVA/3.5MVA Generator with  Primary Controllers/NG Engine Speed & Voltage Control fast/Excitation1/Low Pass Filter 1 / (tr.s +1) (with IC)
      mask TypeOptions FilterType: Lowpass | Highpass
      mask Callback Initialize: p4=get_param(gcb,'Initialize');if strcmp(p4,'on');visible={'on','on','on','on','on','on','on',get_param(gcb,'PlotResponse')};else;visible={'on','on','on','on','off','off','on',get_param(gcb,'PlotResponse')};end;set_param(gcb,'MaskVisibilities',visible)
      mask Callback PlotResponse: p7=get_param(gcb,'PlotResponse');if strcmp(p7,'on');visible={'on','on','on','on',get_param(gcb,'Initialize'),get_param(gcb,'Initialize'),'on','on'};else;visible={'on','on','on','on',get_param(gcb,'Initialize'),get_param(gcb,'Initialize'),'on','off'};end;set_param(gcb,'MaskVisibilities',visible)
      mask Display: plot(X,Y);
  Gain : Gain  Gain=damp(1)/damp(2)  SaturateOnIntegerOverflow=on  OutDataTypeStr=Inherit: Same as input  ParamDataTypeStr=Inherit: Same as input
  Out : Outport
  wires:
  In/1 -> Gain/1
  Gain/1 -> 1st-Order Discrete Filter/1(In)
  1st-Order Discrete Filter/1(Out) -> Out/1

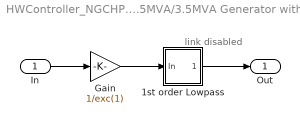
== system HWController_NGCHP_Genset_3p5MVA_lib/HWController_NG_Genset_3.5MVA/3.5MVA Generator with  Primary Controllers/NG Engine Speed & Voltage Control fast/Excitation1/Exciter  1 / (te.s + ke) ==
  note: link disabled
  In : Inport
  1st order Lowpass : Subsystem  AncestorBlock=|  mask(Discrete 1st-Order Filter){FilterType=Lowpass, Tc=exc(2)/exc(1), Ts=Ts, Initialize=on, Vac_Init=[0.0 0 60], Vdc_Init=v0(2), PlotResponse=off, param1=[1 500 0.1]}
      | powerlib_extras/Discrete 
      | Control Blocks/Discrete
      | 1st-Order
      | Discrete Filter
      mask prompts: FilterType "Filter Type:"; Tc "Time constant (s):"; Ts "Sample time:"; Initialize "Initialize filter states"; Vac_Init "AC initial input: [ Mag  Phase(degrees)  Freq(Hz) ]"; Vdc_Init "DC Initial input:"; PlotResponse "Plot filter response"; param1 "Frequency range(Hz) : [Start  End  Inc.]"
      mask init: same as HWController_NGCHP_Genset_3p5MVA_lib/HWController_NG_Genset_3.5MVA/3.5MVA Generator with  Primary Controllers/NG Engine Speed & Voltage Control fast/Excitation1/Low Pass Filter 1 / (tr.s +1) (with IC)
      mask TypeOptions FilterType: Lowpass | Highpass
      mask Callback Initialize: p4=get_param(gcb,'Initialize');if strcmp(p4,'on');visible={'on','on','on','on','on','on','on',get_param(gcb,'PlotResponse')};else;visible={'on','on','on','on','off','off','on',get_param(gcb,'PlotResponse')};end;set_param(gcb,'MaskVisibilities',visible)
      mask Callback PlotResponse: p7=get_param(gcb,'PlotResponse');if strcmp(p7,'on');visible={'on','on','on','on',get_param(gcb,'Initialize'),get_param(gcb,'Initialize'),'on','on'};else;visible={'on','on','on','on',get_param(gcb,'Initialize'),get_param(gcb,'Initialize'),'on','off'};end;set_param(gcb,'MaskVisibilities',visible)
      mask Display: plot(X,Y);
  Gain : Gain  Gain=1/exc(1)  SaturateOnIntegerOverflow=on  OutDataTypeStr=Inherit: Same as input  ParamDataTypeStr=Inherit: Same as input
  Out : Outport
  wires:
  1st order Lowpass/1(Out) -> Out/1
  In/1 -> Gain/1
  Gain/1 -> 1st order Lowpass/1(In)

== system HWController_NGCHP_Genset_3p5MVA_lib/HWController_NG_Genset_3.5MVA/3.5MVA Generator with  Primary Controllers/NG Engine Speed & Voltage Control fast/Excitation1/Lead Lag Compensator tc.s+1 / tb.s+1 ==
  In1 : Inport
  Discrete State-Space : DiscreteStateSpace  A=Ad  B=Bd  C=Cd  D=Dd  X0=x0d  SampleTime=Ts
  Out1 : Outport
  wires:
  Discrete State-Space/1 -> Out1/1
  In1/1 -> Discrete State-Space/1

== system HWController_NGCHP_Genset_3p5MVA_lib/HWController_NG_Genset_3.5MVA/3.5MVA Generator with  Primary Controllers/NG Engine Speed & Voltage Control fast/Excitation1/Low Pass Filter 1 / (tr.s +1) (with IC) ==
  In : Inport
  Discrete State-Space : DiscreteStateSpace  A=Ad  B=Bd  C=Cd  D=Dd  X0=x0d  SampleTime=Ts
  Out : Outport  InitialOutput=0
  wires:
  Discrete State-Space/1 -> Out/1
  In/1 -> Discrete State-Space/1

== system HWController_NGCHP_Genset_3p5MVA_lib/HWController_NG_Genset_3.5MVA/3.5MVA Generator with  Primary Controllers/NG Engine Speed & Voltage Control fast/Excitation1/Main Regulator ka / (ta.s +1) ==
  note: link disabled
  In : Inport
  1st order Lowpass : Subsystem  AncestorBlock=|  mask(Discrete 1st-Order Filter){FilterType=Lowpass, Tc=reg(2), Ts=Ts, Initialize=on, Vac_Init=[0.0 0 60], Vdc_Init=exc(1)*v0(2), PlotResponse=off, param1=[1 500 0.1]}
      | generator_lib/Generator_09222015/GenSet_4MVA_09212015/4MVA Generator with 
      | Primary Controllers1/Diesel Engine
      | Speed & Voltage
      | Control
      | fast/Excitation/Main Regulator
      | ka // (ta.s +1)/1st order
      | Lowpass
      mask prompts: FilterType "Filter Type:"; Tc "Time constant (s):"; Ts "Sample time:"; Initialize "Initialize filter states"; Vac_Init "AC initial input: [ Mag  Phase(degrees)  Freq(Hz) ]"; Vdc_Init "DC Initial input:"; PlotResponse "Plot filter response"; param1 "Frequency range(Hz) : [Start  End  Inc.]"
      mask init: same as HWController_NGCHP_Genset_3p5MVA_lib/HWController_NG_Genset_3.5MVA/3.5MVA Generator with  Primary Controllers/NG Engine Speed & Voltage Control fast/Excitation1/Low Pass Filter 1 / (tr.s +1) (with IC)
      mask TypeOptions FilterType: Lowpass | Highpass
      mask Callback Initialize: p4=get_param(gcb,'Initialize');if strcmp(p4,'on');visible={'on','on','on','on','on','on','on',get_param(gcb,'PlotResponse')};else;visible={'on','on','on','on','off','off','on',get_param(gcb,'PlotResponse')};end;set_param(gcb,'MaskVisibilities',visible)
      mask Callback PlotResponse: p7=get_param(gcb,'PlotResponse');if strcmp(p7,'on');visible={'on','on','on','on',get_param(gcb,'Initialize'),get_param(gcb,'Initialize'),'on','on'};else;visible={'on','on','on','on',get_param(gcb,'Initialize'),get_param(gcb,'Initialize'),'on','off'};end;set_param(gcb,'MaskVisibilities',visible)
      mask Display: plot(X,Y);
  Gain : Gain  Gain=reg(1)  SaturateOnIntegerOverflow=on  OutDataTypeStr=Inherit: Same as input  ParamDataTypeStr=Inherit: Same as input
  Out : Outport
  wires:
  Gain/1 -> 1st order Lowpass/1(In)
  In/1 -> Gain/1
  1st order Lowpass/1(Out) -> Out/1

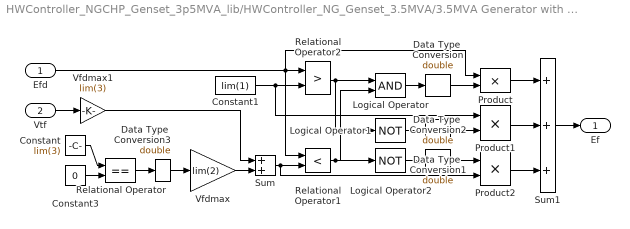
== system HWController_NGCHP_Genset_3p5MVA_lib/HWController_NG_Genset_3.5MVA/3.5MVA Generator with  Primary Controllers/NG Engine Speed & Voltage Control fast/Excitation1/proportional saturation ==
  Efd : Inport
  Vtf : Inport  Port=2
  Constant : Constant  Value=lim(3)
  Constant1 : Constant  Value=lim(1)
  Constant3 : Constant  Value=0
  Data Type  Conversion{,1..3} (4 alike) : DataTypeConversion  OutDataTypeStr=double  SaturateOnIntegerOverflow=on  RndMeth=Zero
  Logical Operator : Logic
  Logical Operator1 : Logic  Operator=NOT  Inputs=1
  Logical Operator2 : Logic  Operator=NOT  Inputs=1
  Product : Product  SaturateOnIntegerOverflow=on  InputSameDT=on  OutDataTypeStr=Inherit: Same as first input
  Product1 : Product  SaturateOnIntegerOverflow=on  InputSameDT=on  OutDataTypeStr=Inherit: Same as first input
  Product2 : Product  SaturateOnIntegerOverflow=on  InputSameDT=on  OutDataTypeStr=Inherit: Same as first input
  Relational Operator : RelationalOperator  Operator===  InputSameDT=on
  Relational Operator1 : RelationalOperator  Operator=<  InputSameDT=on
  Relational Operator2 : RelationalOperator  Operator=>  InputSameDT=on
  Sum : Sum  SaturateOnIntegerOverflow=on  InputSameDT=on  OutDataTypeStr=Inherit: Same as first input
  Sum1 : Sum  Inputs=+++  SaturateOnIntegerOverflow=on  InputSameDT=on  OutDataTypeStr=Inherit: Same as first input
  Vfdmax : Gain  Gain=lim(2)  SaturateOnIntegerOverflow=on  OutDataTypeStr=Inherit: Same as input  ParamDataTypeStr=Inherit: Same as input
  Vfdmax1 : Gain  Gain=lim(3)  SaturateOnIntegerOverflow=on  OutDataTypeStr=Inherit: Same as input  ParamDataTypeStr=Inherit: Same as input
  Ef : Outport  InitialOutput=0
  wires:
  Vtf/1 -> Vfdmax1/1
  Constant/1 -> Relational Operator/1
  Constant3/1 -> Relational Operator/2
  Vfdmax/1 -> Sum/2
  Vfdmax1/1 -> Sum/1
  Sum/1 -> Product2/2, Relational Operator1/2
  Relational Operator2/1 -> Logical Operator1/1, Logical Operator/1
  Relational Operator1/1 -> Logical Operator2/1, Logical Operator/2
  Constant1/1 -> Relational Operator2/2, Product1/1
  Efd/1 -> Relational Operator2/1, Relational Operator1/1, Product/1
  Sum1/1 -> Ef/1
  Product/1 -> Sum1/1
  Product2/1 -> Sum1/3
  Product1/1 -> Sum1/2
  Logical Operator/1 -> Data Type  Conversion/1
  Data Type  Conversion/1 -> Product/2
  Logical Operator1/1 -> Data Type  Conversion1/1
  Data Type  Conversion1/1 -> Product1/2
  Logical Operator2/1 -> Data Type  Conversion2/1
  Data Type  Conversion2/1 -> Product2/1
  Relational Operator/1 -> Data Type  Conversion3/1
  Data Type  Conversion3/1 -> Vfdmax/1

== system HWController_NGCHP_Genset_3p5MVA_lib/HWController_NG_Genset_3.5MVA/3.5MVA Generator with  Primary Controllers/NG Engine Speed & Voltage Control fast/Excitation1/Damping kf.s / (tf.s +1)/1st-Order Discrete Filter ==
  In : Inport
  Discrete State-Space : DiscreteStateSpace  A=Ad  B=Bd  C=Cd  D=Dd  X0=x0d  SampleTime=Ts
  Out : Outport  InitialOutput=0
  wires:
  Discrete State-Space/1 -> Out/1
  In/1 -> Discrete State-Space/1

== system HWController_NGCHP_Genset_3p5MVA_lib/HWController_NG_Genset_3.5MVA/3.5MVA Generator with  Primary Controllers/NG Engine Speed & Voltage Control fast/Excitation1/Exciter  1 / (te.s + ke)/1st order Lowpass ==
  In : Inport
  Discrete State-Space : DiscreteStateSpace  A=Ad  B=Bd  C=Cd  D=Dd  X0=x0d  SampleTime=Ts
  Out : Outport  InitialOutput=0
  wires:
  Discrete State-Space/1 -> Out/1
  In/1 -> Discrete State-Space/1

== system HWController_NGCHP_Genset_3p5MVA_lib/HWController_NG_Genset_3.5MVA/3.5MVA Generator with  Primary Controllers/NG Engine Speed & Voltage Control fast/Excitation1/Main Regulator ka / (ta.s +1)/1st order Lowpass ==
  In : Inport
  Discrete State-Space : DiscreteStateSpace  A=Ad  B=Bd  C=Cd  D=Dd  X0=x0d  SampleTime=Ts
  Out : Outport  InitialOutput=0
  wires:
  Discrete State-Space/1 -> Out/1
  In/1 -> Discrete State-Space/1
